simulink model "problem4"  (R2020b)
settings: Solver=VariableStepAuto  StartTime=0.0  StopTime=10.0  RelTol=1e-3
values from neighbouring files (symbols this model uses):
  b = 3.5077E-6    (= 3.5077e-06)    [prob4.m]    (also in problem4datadic.sldd = 3.5077E-6)
  J = 3.2284E-6    (= 3.2284e-06)    [prob4.m]    (also in problem4datadic.sldd = 3.2284E-6)
  K = 0.0274    [prob4.m]    (also in problem4datadic.sldd)
  Kd = Kd + 0.1    (= 0.15)    [prob4.m]    (also in problem4.m)
  Ki = 100    [prob4.m]    (also in problem4.m)
  Kp = 21    [prob4.m]    (also in problem4.m)
  L = 2.75E-6    (= 2.75e-06)    [prob4.m]    (also in problem4datadic.sldd = 2.75E-6)
  R = 4    [prob4.m]    (also in problem4datadic.sldd = 4.0)
settings Model: DataDictionary=problem4datadic.sldd  Creator=Nitin  LastModifiedBy=Nitin

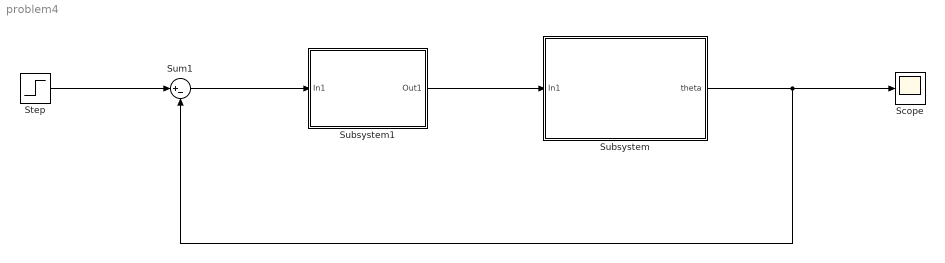
== system problem4 ==
  Scope : Scope
  Step : Step  SampleTime=0
  Subsystem : Subsystem
  Subsystem1 : Subsystem
  Sum1 : Sum  Inputs=|+-
  wires:
  Step/1 -> Sum1/1
  Sum1/1 -> Subsystem1/1(In1)
  Subsystem1/1(Out1) -> Subsystem/1(In1)
  Subsystem/1(theta) -> Scope/1, Sum1/2

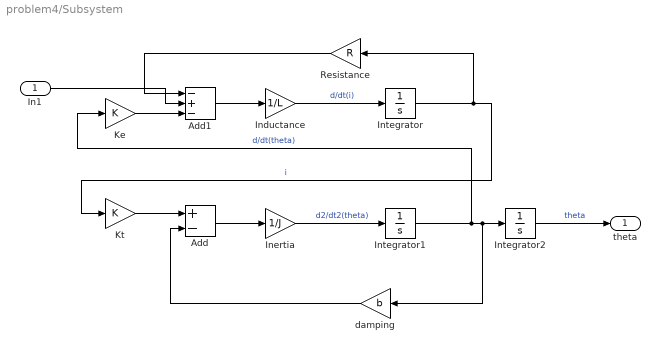
== system problem4/Subsystem ==
  In1 : Inport
  Add : Sum  Inputs=+-
  Add1 : Sum  Inputs=-+-
  Inductance : Gain  Gain=1/L
  Inertia : Gain  Gain=1/J
  Integrator : Integrator
  Integrator1 : Integrator
  Integrator2 : Integrator
  Ke : Gain  Gain=K
  Kt : Gain  Gain=K
  Resistance : Gain  Gain=R
  damping : Gain  Gain=b
  theta : Outport
  wires:
  damping/1 -> Add/2
  Integrator/1 -> Kt/1, Resistance/1  "i"
  In1/1 -> Add1/2
  Add/1 -> Inertia/1
  Add1/1 -> Inductance/1
  Integrator1/1 -> Ke/1, Integrator2/1, damping/1  "d/dt(theta)"
  Inductance/1 -> Integrator/1  "d/dt(i)"
  Integrator2/1 -> theta/1  "theta"
  Inertia/1 -> Integrator1/1  "d2/dt2(theta)"
  Kt/1 -> Add/1
  Resistance/1 -> Add1/1
  Ke/1 -> Add1/3

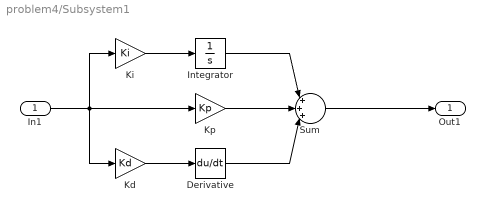
== system problem4/Subsystem1 ==
  In1 : Inport
  Derivative : Derivative
  Integrator : Integrator
  Kd : Gain  Gain=Kd
  Ki : Gain  Gain=Ki
  Kp : Gain  Gain=Kp
  Sum : Sum  Inputs=|+++|
  Out1 : Outport
  wires:
  Derivative/1 -> Sum/3
  In1/1 -> Kd/1, Ki/1, Kp/1
  Kd/1 -> Derivative/1
  Ki/1 -> Integrator/1
  Integrator/1 -> Sum/1
  Kp/1 -> Sum/2
  Sum/1 -> Out1/1
